simulink model "MedianFilter"  (R2018b)
settings: Solver=FixedStepAuto  StartTime=0.0  StopTime=1  FixedStep=1  RelTol=1e-3
model workspace (MAT data in the model file):
  SL_ROS_VariableLengthArrays_MaxSizes.CommonInfo.ArrayTruncateAction = 'EmitWarning'
  SL_ROS_VariableLengthArrays_MaxSizes.MsgTypeMap = containers.Map
  SL_ROS_VariableLengthArrays_MaxSizes.MsgTypeMap.serialization.keys = {'sensor_msgs/Image'}
  SL_ROS_VariableLengthArrays_MaxSizes.MsgTypeMap.serialization.values{1}(1).PropertyName = 'Data'
  SL_ROS_VariableLengthArrays_MaxSizes.MsgTypeMap.serialization.values{1}(1).DataType = 'uint8'
  SL_ROS_VariableLengthArrays_MaxSizes.MsgTypeMap.serialization.values{1}(1).MaxLength = 4147200
  SL_ROS_VariableLengthArrays_MaxSizes.MsgTypeMap.serialization.values{1}(2).PropertyName = 'Encoding'
  SL_ROS_VariableLengthArrays_MaxSizes.MsgTypeMap.serialization.values{1}(2).DataType = 'uint8'
  SL_ROS_VariableLengthArrays_MaxSizes.MsgTypeMap.serialization.values{1}(2).MaxLength = 4147200
  SL_ROS_VariableLengthArrays_MaxSizes.MsgTypeMap.serialization.uniformity = 0
  SL_ROS_VariableLengthArrays_MaxSizes.MsgTypeMap.serialization.keyType = 'char'
  SL_ROS_VariableLengthArrays_MaxSizes.MsgTypeMap.serialization.valueType = 'any'
undefined symbols (not defined in the file or in its folder): a
libraries: svdutilitieslib x3, visionanalysis x1
settings Model: Creator=HannesDittmann  LastModifiedBy=HannesDittmann
settings DebuggingCC: UnderSpecifiedDimensionMsg=warning

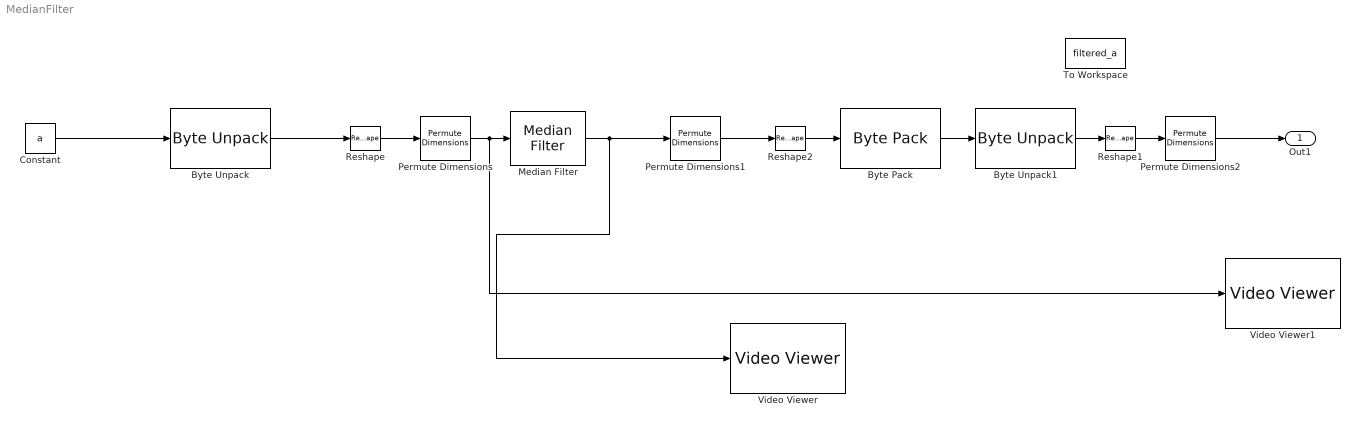
== system MedianFilter ==
  Byte Pack : svdutilitieslib/Byte Pack  maskPackedDataType=uint8  datatypes={'uint16'}  byteAlign=1  blockPlatform=arduinoert
      settings: SourceProductName=Simulink Support Package for Arduino Hardware  SourceProductBaseCode=ARDUINO
  Byte Unpack : svdutilitieslib/Byte Unpack  dimensions={[2073600]}  datatypes={'uint16'}  byteAlign=1  blockPlatform=arduinoert
      settings: SourceProductName=Simulink Support Package for Arduino Hardware  SourceProductBaseCode=ARDUINO
  Byte Unpack1 : svdutilitieslib/Byte Unpack  dimensions={[2073600]}  datatypes={'uint16'}  byteAlign=1  blockPlatform=arduinoert
      settings: SourceProductName=Simulink Support Package for Arduino Hardware  SourceProductBaseCode=ARDUINO
  Constant : Constant  Value=a
  Median Filter : visionanalysis/Median Filter  nghbood=[10]  outSize=Same as input port I  padType=Symmetric  padSrc=Specify via dialog  padVal=0  roundingMode=Floor  overflowMode=off
      settings: SourceProductName=Computer Vision System Toolbox  SourceProductBaseCode=VP
  Permute Dimensions : PermuteDimensions
  Permute Dimensions1 : PermuteDimensions
  Permute Dimensions2 : PermuteDimensions
  Reshape : Reshape  OutputDimensionality=Customize  OutputDimensions=[1920,1080]
  Reshape1 : Reshape  OutputDimensionality=Customize  OutputDimensions=[1920,1080]
  Reshape2 : Reshape  OutputDimensions=[1920,1080]
  To Workspace : ToWorkspace  VariableName=filtered_a  SampleTime=-1
  Video Viewer : VideoViewer  FigPos=[1 1030 1280 630]
  Video Viewer1 : VideoViewer  FigPos=[1 1030 1680 880]
  Out1 : Outport
  wires:
  Constant/1 -> Byte Unpack/1
  Byte Unpack/1 -> Reshape/1
  Reshape/1 -> Permute Dimensions/1
  Permute Dimensions/1 -> Video Viewer1/1, Median Filter/1
  Byte Unpack1/1 -> Reshape1/1
  Reshape1/1 -> Permute Dimensions2/1
  Median Filter/1 -> Video Viewer/1, Permute Dimensions1/1
  Permute Dimensions2/1 -> Out1/1
  Permute Dimensions1/1 -> Reshape2/1
  Reshape2/1 -> Byte Pack/1
  Byte Pack/1 -> Byte Unpack1/1
